simulink model "orbit_dynamics"  (R2023b)
settings: Solver=FixedStepAuto  StartTime=0.0  StopTime=1000.0  FixedStep=0.001  RelTol=1e-3
InitFcn:
  | load('orbit_dynamics_initial.mat')
undefined symbols (not defined in the file or in its folder): m
settings Model: SimulationMode=rapid-accelerator  Creator=orous  LastModifiedBy=xlxs4
settings DataIOCC: ExternalInput=f_in  LoadExternalInput=on

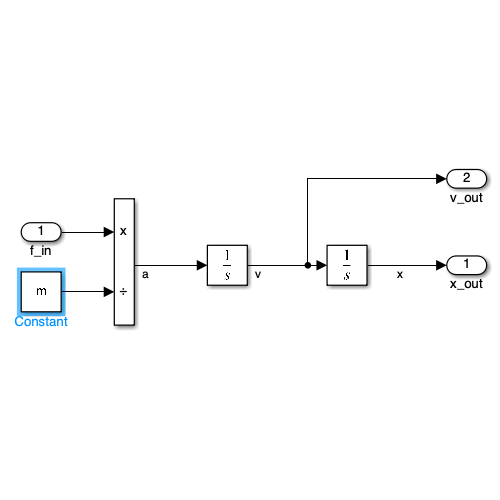
[thumbnail: Simulink's stored preview of the top-level diagram]
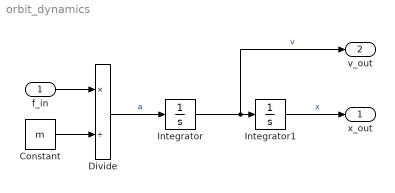
== system orbit_dynamics ==
  f_in : Inport  Unit=N  PortDimensions=3
  Constant : Constant  Value=m
  Divide : Product  Inputs=*/
  Integrator : Integrator
  Integrator1 : Integrator
  x_out : Outport
  v_out : Outport  Port=2
  wires:
  f_in/1 -> Divide/1
  Constant/1 -> Divide/2
  Divide/1 -> Integrator/1  "a"
  Integrator/1 -> v_out/1, Integrator1/1  "v"
  Integrator1/1 -> x_out/1  "x"
